simulink model "whirlybirdsim"  (R2013a)
settings: Solver=ode45  StartTime=0.0  StopTime=100  RelTol=1e-3
InitFcn:
  | param
values from neighbouring files (symbols this model uses):
  P = defineParameters    [plotWhirlybird.m]
undefined symbols (not defined in the file or in its folder): autopilot, plotWhirlybird, plotwhirlybirdstatevariables
libraries: simulink x2
settings Model: Creator=Administrator  LastModifiedBy=beard
settings DataIOCC: SignalLoggingSaveFormat=ModelDataLogs
settings OptimizationCC: ExpressionDepthLimit=2147483647
settings DebuggingCC: FcnCallInpInsideContextMsg=UseLocalSettings  StrictBusMsg=Warning
settings GRTTargetCC: CombineOutputUpdateFcns=off  GRTInterface=on

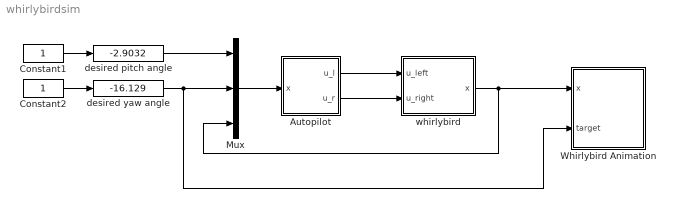
== system whirlybirdsim ==
  Autopilot : Subsystem
  Constant1 : Constant
  Constant2 : Constant
  Mux : Mux  Inputs=3
  Whirlybird Animation : Subsystem
      mask Display: image(imread('tv.jpg'))
  desired pitch angle : simulink/Math Operations/Slider Gain  low=-30  gain=-2.9032  high=30
  desired yaw angle : simulink/Math Operations/Slider Gain  low=-100  gain=-16.129  high=100
  whirlybird : Subsystem
      mask Display: image(imread('whirlybird.jpg'))
  wires:
  Autopilot/1(u_l) -> whirlybird/1(u_left)
  whirlybird/1(x) -> Whirlybird Animation/1(x), Mux/3
  Mux/1 -> Autopilot/1(x)
  Constant1/1 -> desired pitch angle/1
  desired pitch angle/1 -> Mux/1
  Constant2/1 -> desired yaw angle/1
  desired yaw angle/1 -> Mux/2, Whirlybird Animation/2(target)
  Autopilot/2(u_r) -> whirlybird/2(u_right)

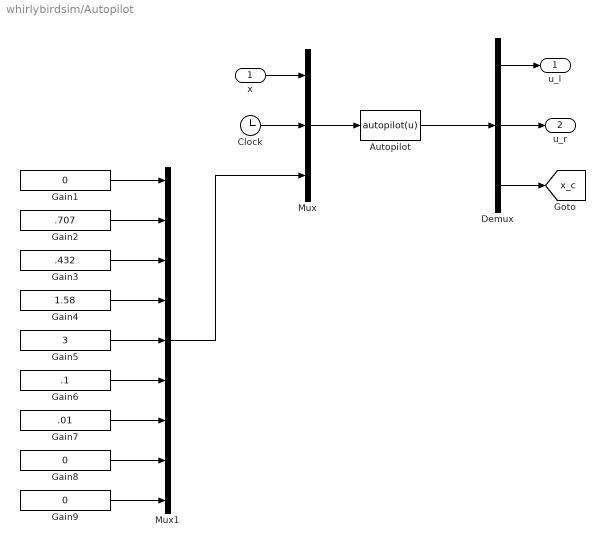
== system whirlybirdsim/Autopilot ==
  x : Inport
  Autopilot : MATLABFcn  MATLABFcn=autopilot(u)  OutputDimensions=2+10  SampleTime=P.Ts
  Clock : Clock
  Demux : Demux  Outputs=[1;1;10]
  Gain1 : Constant  Value=0  VectorParams1D=off
  Gain2 : Constant  Value=.707  VectorParams1D=off
  Gain3 : Constant  Value=.432  VectorParams1D=off
  Gain4 : Constant  Value=1.58  VectorParams1D=off
  Gain5 : Constant  Value=3  VectorParams1D=off
  Gain6 : Constant  Value=.1  VectorParams1D=off
  Gain7 : Constant  Value=.01  VectorParams1D=off
  Gain8 : Constant  Value=0  VectorParams1D=off
  Gain9 : Constant  Value=0  VectorParams1D=off
  Mux : Mux  Inputs=3
  Mux1 : Mux  Inputs=9
  u_l : Outport
  u_r : Outport  Port=2
  tag scope: x_c=global
  wires:
  Mux/1 -> Autopilot/1
  x/1 -> Mux/1
  Clock/1 -> Mux/2
  Demux/1 -> u_l/1
  Autopilot/1 -> Demux/1
  Demux/2 -> u_r/1
  Demux/3 -> [x_c]
  Mux1/1 -> Mux/3
  Gain1/1 -> Mux1/1
  Gain2/1 -> Mux1/2
  Gain3/1 -> Mux1/3
  Gain4/1 -> Mux1/4
  Gain5/1 -> Mux1/5
  Gain6/1 -> Mux1/6
  Gain7/1 -> Mux1/7
  Gain8/1 -> Mux1/8
  Gain9/1 -> Mux1/9

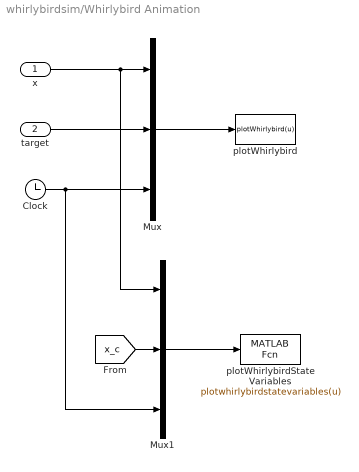
== system whirlybirdsim/Whirlybird Animation ==
  x : Inport
  target : Inport  Port=2
  Clock : Clock
  Mux : Mux  Inputs=3
  Mux1 : Mux  Inputs=3
  plotWhirlybird : MATLABFcn  MATLABFcn=plotWhirlybird(u)  OutputDimensions=0  SampleTime=0.1
  plotWhirlybirdState Variables : MATLABFcn  MATLABFcn=plotwhirlybirdstatevariables(u)  OutputDimensions=0  SampleTime=0.1
  wires:
  Clock/1 -> Mux/3, Mux1/3
  x/1 -> Mux/1, Mux1/1
  Mux/1 -> plotWhirlybird/1
  target/1 -> Mux/2
  [x_c] -> Mux1/2
  Mux1/1 -> plotWhirlybirdState Variables/1

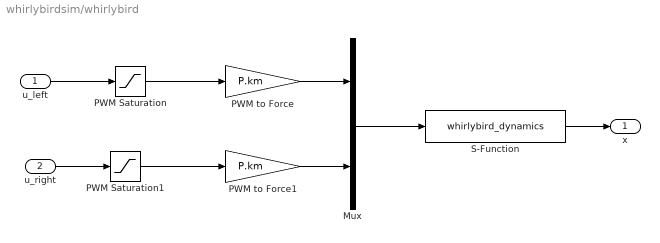
== system whirlybirdsim/whirlybird ==
  u_left : Inport
  u_right : Inport  Port=2
  Mux : Mux  Inputs=2
  PWM Saturation : Saturate  UpperLimit=100  LowerLimit=0
  PWM Saturation1 : Saturate  UpperLimit=100  LowerLimit=0
  PWM to Force : Gain  Gain=P.km
  PWM to Force1 : Gain  Gain=P.km
  S-Function : S-Function  FunctionName=whirlybird_dynamics  Parameters=P  EnableBusSupport=off
  x : Outport
  wires:
  S-Function/1 -> x/1
  Mux/1 -> S-Function/1
  PWM to Force/1 -> Mux/1
  PWM Saturation/1 -> PWM to Force/1
  u_left/1 -> PWM Saturation/1
  u_right/1 -> PWM Saturation1/1
  PWM to Force1/1 -> Mux/2
  PWM Saturation1/1 -> PWM to Force1/1
